simulink model "voltage_measure"  (R2025b)
settings: Solver=ode1be  StartTime=0.0  StopTime=simlength  FixedStep=ts  RelTol=1e-3
undefined symbols (not defined in the file): ts
libraries: fl_lib x36, nesl_utility x11, ee_lib x2, simulink x1
settings Model: Creator=ltnbda  LastModifiedBy=dbagn
settings DataIOCC: SaveOutput=off  SignalLogging=off  DSMLogging=off  SaveTime=off  ReturnWorkspaceOutputs=off
settings RTWCC: GPUComputeCapability=3.5

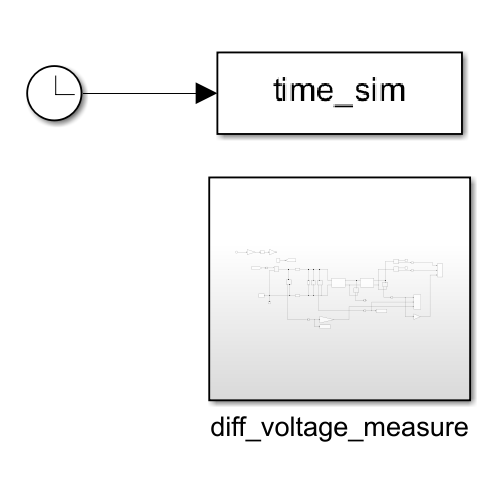
[thumbnail: Simulink's stored preview of the top-level diagram]
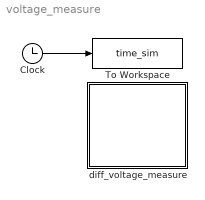
== system voltage_measure ==
  Clock : Clock
  To Workspace : ToWorkspace  VariableName=time_sim  SampleTime=ts
      settings: MaxDataPoints=N  Save2DSignal=2-D array (concatenate along first dimension)
  diff_voltage_measure : Subsystem
  wires:
  Clock/1 -> To Workspace/1

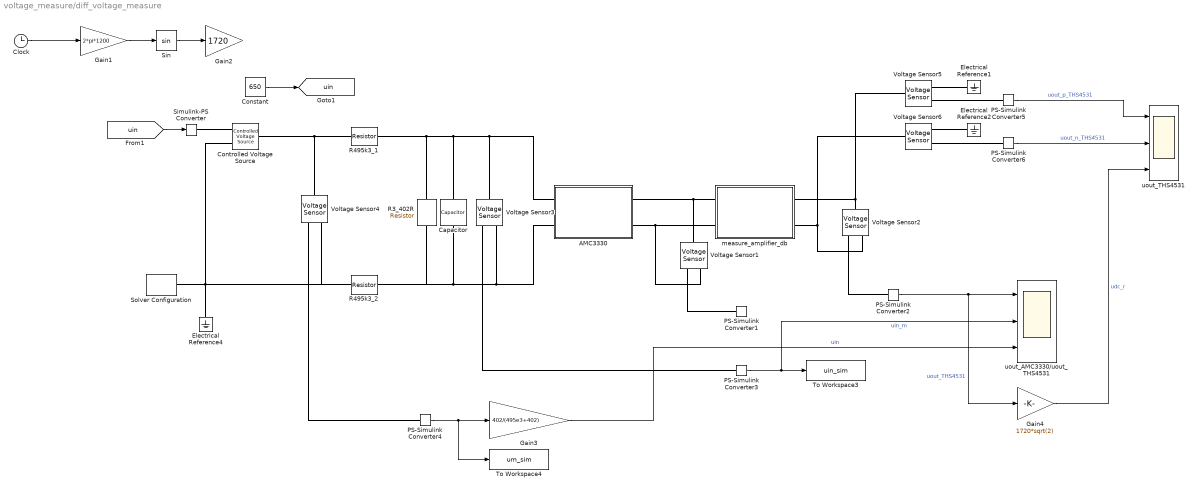
== system voltage_measure/diff_voltage_measure ==
  AMC3330 : Subsystem
  Capacitor : fl_lib/Electrical/Electrical Elements/Capacitor  c=0.1e-6 F  r=1e-6 Ohm  g=0 1/Ohm  i_specify=off  i_priority=None  i=0 A  i_nominal_specify=off  i_nominal_value=1  i_nominal_unit=A  v_specify=off  v_priority=None  v=0 V  v_nominal_specify=off  v_nominal_value=1  v_nominal_unit=V  vc_specify=off  vc_priority=High  vc=0 V  vc_nominal_specify=off  vc_nominal_value=1  vc_nominal_unit=V
  Clock : Clock
  Constant : Constant  Value=650
  Controlled Voltage Source : fl_lib/Electrical/Electrical Sources/Controlled Voltage Source
  Electrical Reference1 : fl_lib/Electrical/Electrical Elements/Electrical Reference
  Electrical Reference2 : fl_lib/Electrical/Electrical Elements/Electrical Reference
  Electrical Reference4 : fl_lib/Electrical/Electrical Elements/Electrical Reference
  Gain1 : Gain  Gain=2*pi*1200
  Gain2 : Gain  Gain=1720
  Gain3 : Gain  Gain=402/(495e3+402)
  Gain4 : Gain  Gain=1720*sqrt(2)
  PS-Simulink Converter{1..6} (6 alike) : nesl_utility/PS-Simulink Converter  PhysicalDomain=network_engine_domain  SubClassName=ps_output  LeftPortType=input  RightPortType=output  PseudoPeriodic=off  Frequencies=[]  VectorFormat=1-D array  Unit=V  AffineConversion=off
  R3_402R : fl_lib/Electrical/Electrical Elements/Resistor  R=402 Ohm  i_specify=off  i_priority=None  i=0 A  i_nominal_specify=off  i_nominal_value=1  i_nominal_unit=A  v_specify=off  v_priority=None  v=0 V  v_nominal_specify=off  v_nominal_value=1  v_nominal_unit=V
  R495k3_1 : fl_lib/Electrical/Electrical Elements/Resistor  R=400e3+95.3e3 Ohm  i_specify=off  i_priority=None  i=0 A  i_nominal_specify=off  i_nominal_value=1  i_nominal_unit=A  v_specify=off  v_priority=None  v=0 V  v_nominal_specify=off  v_nominal_value=1  v_nominal_unit=V
  R495k3_2 : fl_lib/Electrical/Electrical Elements/Resistor  R=400e3+95.3e3 Ohm  i_specify=off  i_priority=None  i=0 A  i_nominal_specify=off  i_nominal_value=1  i_nominal_unit=A  v_specify=off  v_priority=None  v=0 V  v_nominal_specify=off  v_nominal_value=1  v_nominal_unit=V
  Simulink-PS Converter : nesl_utility/Simulink-PS Converter  PhysicalDomain=network_engine_domain  SubClassName=ps_input  LeftPortType=input  RightPortType=output  PseudoPeriodic=off  Frequencies=[]  NoiseDistribution=none  NoiseParameters=[]  Unit=V  AffineConversion=off  FilteringAndDerivatives=provide  SimscapeFilterOrder=1  InputFilterTimeConstant=0.001  UdotUserProvided=0
  Sin : Trigonometry
  Solver Configuration : nesl_utility/Solver Configuration  PhysicalDomain=network_engine_domain  SubClassName=solver  LeftPortType=input  RightPortType=generic  Tones=[]  Harmonics=[]  SimulateNoise=off  Profile=off  UseLocalSampling=off  EnableSwitchedLinearOptims=on  FrequencyDomain=off  UseCCode=off  RelTol=0.001  AbsTol=0.001  MinStep=1e-09  ToWorkspace=off  RevertToSquareIcSolve=off  NumHomotopyIterations=100  PhasorMode=off  PhasorModeNumHarmonics=1  ConsistencySolver=NEWTON_XTOL_AFTER_FTOL  IndexReductionMethod=DerivativeReplacement  DoDC=on  ResidualTolerance=1e-09  ConsistencyTolSource=GLOBAL  ConsistencyAbsTol=0.001  ConsistencyRelTol=0.001  ConsistencyTolFactor=0.001  UseLocalSolver=on  LocalSolverChoice=NE_BACKWARD_EULER_ADVANCER  ResolveIndetEquations=on  FunctionEvalNumThread=1  LocalSolverSampleTime=ts  DoFixedCost=on  MaxNonlinIter=3  MaxModeIter=2  ComputeImpulses=off  ImpulseIterations=2  LinearAlgebra=auto  LinearAlgebraNumThread=0  EquationFormulation=NE_TIME_EF  DelaysMemoryBudget=1024  AutomaticFiltering=on  FilteringTimeConstant=0.001  PartitionStorageMethod=AS_NEEDED  PartitionMemoryBudget=1024  PartitionMethod=ROBUST  MultibodyUseLocalSolver=off  MultibodyLocalSolverChoice=ODE1  MultibodyLocalSolverSampleTime=0.001
  To Workspace3 : ToWorkspace  VariableName=uin_sim  SampleTime=ts
      settings: MaxDataPoints=N  Save2DSignal=2-D array (concatenate along first dimension)
  To Workspace4 : ToWorkspace  VariableName=um_sim  SampleTime=ts
      settings: MaxDataPoints=N  Save2DSignal=2-D array (concatenate along first dimension)
  Voltage Sensor{1..6} (6 alike) : fl_lib/Electrical/Electrical Sensors/Voltage Sensor
  measure_amplifier_db : Subsystem
  uout_AMC3330/uout_THS4531 : Scope  NumInputPorts=3
      settings: SampleTime=ts  ActiveDisplayYMinimum=0.26272599465267665  ActiveDisplayYMaximum=0.26382578383618316  DataLoggingVariableName=ScopeData2
  uout_THS4531 : Scope  NumInputPorts=3
      settings: ActiveDisplayString=3  ActiveDisplayYMinimum=582.121734260681  ActiveDisplayYMaximum=701.68902969605745  DataLoggingVariableName=ScopeData4
  tag scope: uin=global
  wires:
  PS-Simulink Converter2/1 -> uout_AMC3330/uout_THS4531/1, Gain4/1  "uout_THS4531"
  PS-Simulink Converter3/1 -> uout_AMC3330/uout_THS4531/2, To Workspace3/1  "uin_m"
  PS-Simulink Converter4/1 -> Gain3/1, To Workspace4/1
  [uin] -> Simulink-PS Converter/1
  Sin/1 -> Gain2/1
  Clock/1 -> Gain1/1
  Gain1/1 -> Sin/1
  Constant/1 -> [uin]
  PS-Simulink Converter5/1 -> uout_THS4531/1  "uout_p_THS4531"
  PS-Simulink Converter6/1 -> uout_THS4531/2  "uout_n_THS4531"
  Gain3/1 -> uout_AMC3330/uout_THS4531/3  "uin"
  Gain4/1 -> uout_THS4531/3  "udc_r"
  connections:
  R495k3_2/LConn1 -- Voltage Sensor4/RConn2 -- Controlled Voltage Source/RConn2 -- Solver Configuration/RConn1 -- Electrical Reference4/LConn1
  Controlled Voltage Source/LConn1 -- Voltage Sensor4/LConn1 -- R495k3_1/LConn1
  Simulink-PS Converter/RConn1 -- Controlled Voltage Source/RConn1
  R3_402R/LConn1 -- R495k3_1/RConn1 -- Capacitor/LConn1 -- Voltage Sensor3/LConn1 -- AMC3330/LConn1
  R495k3_2/RConn1 -- R3_402R/RConn1 -- Capacitor/RConn1 -- Voltage Sensor3/RConn2 -- AMC3330/LConn2
  AMC3330/RConn1 -- measure_amplifier_db/LConn1 -- Voltage Sensor1/LConn1
  Voltage Sensor2/LConn1 -- Voltage Sensor5/LConn1 -- measure_amplifier_db/RConn1
  Voltage Sensor2/RConn1 -- PS-Simulink Converter2/LConn1
  AMC3330/RConn2 -- Voltage Sensor1/RConn2 -- measure_amplifier_db/LConn2
  Voltage Sensor2/RConn2 -- Voltage Sensor6/LConn1 -- measure_amplifier_db/RConn2
  PS-Simulink Converter4/LConn1 -- Voltage Sensor4/RConn1
  Voltage Sensor3/RConn1 -- PS-Simulink Converter3/LConn1
  Voltage Sensor1/RConn1 -- PS-Simulink Converter1/LConn1
  Electrical Reference1/LConn1 -- Voltage Sensor5/RConn2
  Electrical Reference2/LConn1 -- Voltage Sensor6/RConn2
  PS-Simulink Converter5/LConn1 -- Voltage Sensor5/RConn1
  Voltage Sensor6/RConn1 -- PS-Simulink Converter6/LConn1

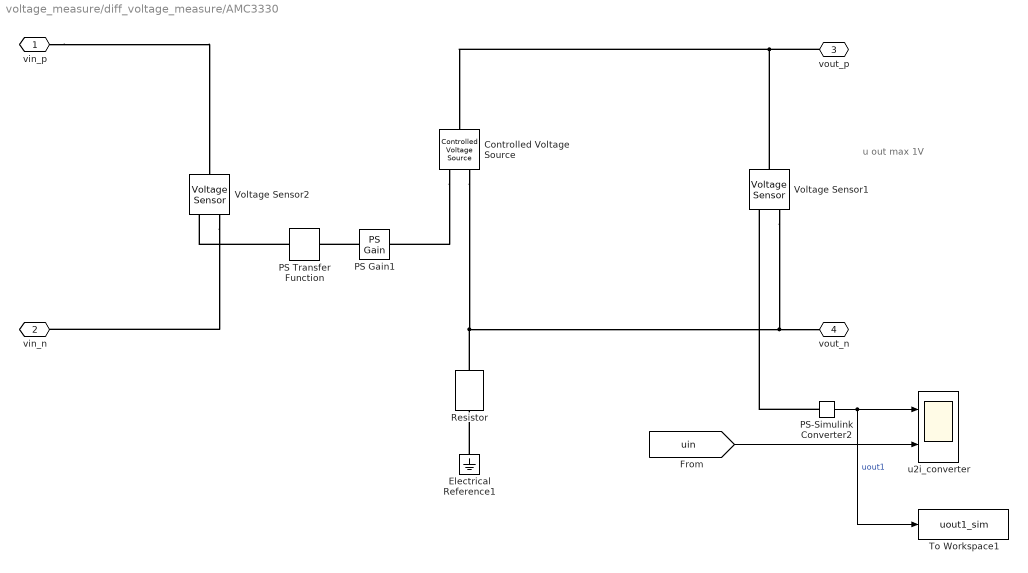
== system voltage_measure/diff_voltage_measure/AMC3330 ==
  note: u out max 1V
  Controlled Voltage Source : fl_lib/Electrical/Electrical Sources/Controlled Voltage Source
  Electrical Reference1 : fl_lib/Electrical/Electrical Elements/Electrical Reference
  PS Gain1 : fl_lib/Physical Signals/Functions/PS Gain  gain=2
  PS Transfer Function : fl_lib/Physical Signals/Linear Operators/PS Transfer Function  transfer_function_type=foundation.enum.transfer_function_type.lag  T=ts s  T1=2 s  T2=1 s  reset_method=foundation.enum.IntegratorResetSpec.None  initial_condition_spec=foundation.enum.IntegratorICSpec.Internal  y0=0 V
      settings: InternalSimscapePortConfiguration="{\"Bottom\":[],\"Left\":[{\"id\":\"U\",\"label\":\"\",\"type\":\"input\"}],\"Right\":[{\"id\":\"Y\",\"label\":\"\",\"type\":\"output\"}],\"Top\":[]}"
  PS-Simulink Converter2 : nesl_utility/PS-Simulink Converter  PhysicalDomain=network_engine_domain  SubClassName=ps_output  LeftPortType=input  RightPortType=output  PseudoPeriodic=off  Frequencies=[]  VectorFormat=1-D array  Unit=V  AffineConversion=off
  Resistor : fl_lib/Electrical/Electrical Elements/Resistor  R=1e6 Ohm  i_specify=off  i_priority=None  i=0 A  i_nominal_specify=off  i_nominal_value=1  i_nominal_unit=A  v_specify=off  v_priority=None  v=0 V  v_nominal_specify=off  v_nominal_value=1  v_nominal_unit=V
  To Workspace1 : ToWorkspace  VariableName=uout1_sim  SampleTime=ts
      settings: MaxDataPoints=N  Save2DSignal=2-D array (concatenate along first dimension)
  Voltage Sensor1 : fl_lib/Electrical/Electrical Sensors/Voltage Sensor
  Voltage Sensor2 : fl_lib/Electrical/Electrical Sensors/Voltage Sensor
  u2i_converter : Scope  NumInputPorts=2
      settings: SampleTime=ts  ActiveDisplayYMinimum=0.52734505076655569  ActiveDisplayYMaximum=0.52734505076682436
  vin_p : PMIOPort  Side=Left
  vin_n : PMIOPort  Port=2  Side=Left
  vout_p : PMIOPort  Port=3  Side=Right
  vout_n : PMIOPort  Port=4  Side=Right
  wires:
  [uin] -> u2i_converter/2
  PS-Simulink Converter2/1 -> To Workspace1/1, u2i_converter/1  "uout1"
  connections:
  vin_p/RConn1 -- Voltage Sensor2/LConn1
  Voltage Sensor2/RConn2 -- vin_n/RConn1
  PS Transfer Function/LConn1 -- Voltage Sensor2/RConn1
  Controlled Voltage Source/RConn1 -- PS Gain1/RConn1
  vout_p/RConn1 -- Controlled Voltage Source/LConn1 -- Voltage Sensor1/LConn1
  Controlled Voltage Source/RConn2 -- Resistor/LConn1 -- Voltage Sensor1/RConn2 -- vout_n/RConn1
  PS Gain1/LConn1 -- PS Transfer Function/RConn1
  PS-Simulink Converter2/LConn1 -- Voltage Sensor1/RConn1
  Electrical Reference1/LConn1 -- Resistor/RConn1

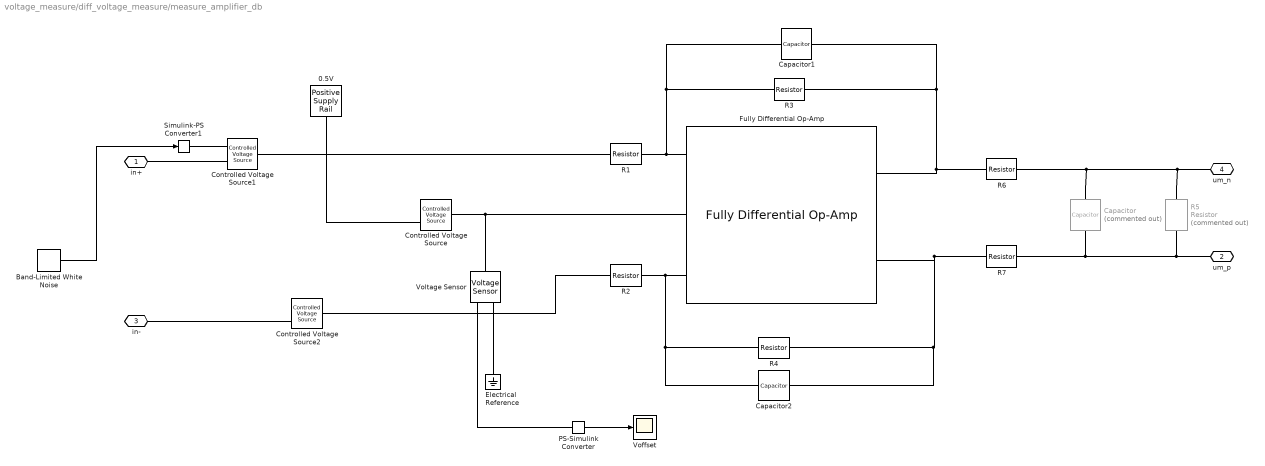
== system voltage_measure/diff_voltage_measure/measure_amplifier_db ==
  0.5V : ee_lib/Sources/Positive Supply Rail  v0=0.5 V
      settings: InternalSimscapePortConfiguration="{\"Bottom\":[],\"Left\":[],\"Right\":[{\"id\":\"p\",\"label\":\"\",\"type\":\"foundation.electrical.electrical\"}],\"Top\":[]}"
  Band-Limited White Noise : simulink/Sources/Band-Limited White Noise  Cov=1e-9  Ts=ts  seed=[23341]
  Capacitor : fl_lib/Electrical/Electrical Elements/Capacitor  Commented=on  c=22e-9 F  r=1e-6 Ohm  g=0 1/Ohm  i_specify=off  i_priority=None  i=0 A  i_nominal_specify=off  i_nominal_value=1  i_nominal_unit=A  v_specify=off  v_priority=None  v=0 V  v_nominal_specify=off  v_nominal_value=1  v_nominal_unit=V  vc_specify=off  vc_priority=High  vc=0 V  vc_nominal_specify=off  vc_nominal_value=1  vc_nominal_unit=V
  Capacitor1 : fl_lib/Electrical/Electrical Elements/Capacitor  c=5e-9 F  r=1e-6 Ohm  g=0 1/Ohm  i_specify=off  i_priority=None  i=0 A  i_nominal_specify=off  i_nominal_value=1  i_nominal_unit=A  v_specify=off  v_priority=None  v=0 V  v_nominal_specify=off  v_nominal_value=1  v_nominal_unit=V  vc_specify=off  vc_priority=High  vc=0 V  vc_nominal_specify=off  vc_nominal_value=1  vc_nominal_unit=V
  Capacitor2 : fl_lib/Electrical/Electrical Elements/Capacitor  c=5e-9 F  r=1e-6 Ohm  g=0 1/Ohm  i_specify=off  i_priority=None  i=0 A  i_nominal_specify=off  i_nominal_value=1  i_nominal_unit=A  v_specify=off  v_priority=None  v=0 V  v_nominal_specify=off  v_nominal_value=1  v_nominal_unit=V  vc_specify=off  vc_priority=High  vc=0 V  vc_nominal_specify=off  vc_nominal_value=1  vc_nominal_unit=V
  Controlled Voltage Source : fl_lib/Electrical/Electrical Sources/Controlled Voltage Source
  Controlled Voltage Source1 : fl_lib/Electrical/Electrical Sources/Controlled Voltage Source
  Controlled Voltage Source2 : fl_lib/Electrical/Electrical Sources/Controlled Voltage Source
  Electrical Reference : fl_lib/Electrical/Electrical Elements/Electrical Reference
  Fully Differential Op-Amp : ee_lib/Integrated Circuits/Fully Differential Op-Amp  A=1e3  f=1.5 GHz  Rdiff=1.3 MOhm  Cdiff=1.8 pF  Rcom=1.0 MOhm  Ccom=2.3 pF  Rout=1 Ohm  Vmin=-1.4 V  Vmax=1.4 V  Vdotdiff=5000 V/us  Rocm=23.0 kOhm  Vs_neg=-5 V  Vs_pos=5 V  V0=0 V
      settings: InternalSimscapePortConfiguration="{\"Bottom\":[],\"Left\":[{\"id\":\"n\",\"label\":\"-\",\"type\":\"foundation.electrical.electrical\"},{\"id\":\"cm\",\"label\":\"cm\",\"type\":\"foundation.electrical.electrical\"},{\"id\":\"p\",\"label\":\"+\",\"type\":\"foundation.electrical.electrical\"}],\"Right\":[{\"id\":\"out_p\",\"label\":\"+\",\"type\":\"foundation.electrical.electrical\"},{\"id\":\"out_n\",\"label\":\"-\",\"type\":\"foundation.electrical.electrical\"}],\"Top\":[]}"
  PS-Simulink Converter : nesl_utility/PS-Simulink Converter  PhysicalDomain=network_engine_domain  SubClassName=ps_output  LeftPortType=input  RightPortType=output  PseudoPeriodic=off  Frequencies=[]  VectorFormat=1-D array  Unit=V  AffineConversion=off
  R1 : fl_lib/Electrical/Electrical Elements/Resistor  R=2e3 Ohm  i_specify=off  i_priority=None  i=0 A  i_nominal_specify=off  i_nominal_value=1  i_nominal_unit=A  v_specify=off  v_priority=None  v=0 V  v_nominal_specify=off  v_nominal_value=1  v_nominal_unit=V
  R2 : fl_lib/Electrical/Electrical Elements/Resistor  R=2e3 Ohm  i_specify=off  i_priority=None  i=0 A  i_nominal_specify=off  i_nominal_value=1  i_nominal_unit=A  v_specify=off  v_priority=None  v=0 V  v_nominal_specify=off  v_nominal_value=1  v_nominal_unit=V
  R3 : fl_lib/Electrical/Electrical Elements/Resistor  R=1e3 Ohm  i_specify=off  i_priority=None  i=0 A  i_nominal_specify=off  i_nominal_value=1  i_nominal_unit=A  v_specify=off  v_priority=None  v=0 V  v_nominal_specify=off  v_nominal_value=1  v_nominal_unit=V
  R4 : fl_lib/Electrical/Electrical Elements/Resistor  R=1e3 Ohm  i_specify=off  i_priority=None  i=0 A  i_nominal_specify=off  i_nominal_value=1  i_nominal_unit=A  v_specify=off  v_priority=None  v=0 V  v_nominal_specify=off  v_nominal_value=1  v_nominal_unit=V
  R5 : fl_lib/Electrical/Electrical Elements/Resistor  Commented=on  R=2e3 Ohm  i_specify=off  i_priority=None  i=0 A  i_nominal_specify=off  i_nominal_value=1  i_nominal_unit=A  v_specify=off  v_priority=None  v=0 V  v_nominal_specify=off  v_nominal_value=1  v_nominal_unit=V
  R6 : fl_lib/Electrical/Electrical Elements/Resistor  R=150 Ohm  i_specify=off  i_priority=None  i=0 A  i_nominal_specify=off  i_nominal_value=1  i_nominal_unit=A  v_specify=off  v_priority=None  v=0 V  v_nominal_specify=off  v_nominal_value=1  v_nominal_unit=V
  R7 : fl_lib/Electrical/Electrical Elements/Resistor  R=150 Ohm  i_specify=off  i_priority=None  i=0 A  i_nominal_specify=off  i_nominal_value=1  i_nominal_unit=A  v_specify=off  v_priority=None  v=0 V  v_nominal_specify=off  v_nominal_value=1  v_nominal_unit=V
  Simulink-PS Converter1 : nesl_utility/Simulink-PS Converter  PhysicalDomain=network_engine_domain  SubClassName=ps_input  LeftPortType=input  RightPortType=output  PseudoPeriodic=off  Frequencies=[]  NoiseDistribution=none  NoiseParameters=[]  Unit=V  AffineConversion=off  FilteringAndDerivatives=provide  SimscapeFilterOrder=1  InputFilterTimeConstant=0.001  UdotUserProvided=0
  Voffset : Scope
      settings: SampleTime=ts  ActiveDisplayYMinimum=-0.059473389598419614  ActiveDisplayYMaximum=1.0507912739067826
  Voltage Sensor : fl_lib/Electrical/Electrical Sensors/Voltage Sensor
  in+ : PMIOPort  Side=Left
  um_p : PMIOPort  Port=2  Side=Right
  in- : PMIOPort  Port=3  Side=Left
  um_n : PMIOPort  Port=4  Side=Right
  wires:
  Band-Limited White Noise/1 -> Simulink-PS Converter1/1
  PS-Simulink Converter/1 -> Voffset/1
  connections:
  R3/RConn1 -- Capacitor1/RConn1 -- R6/LConn1 -- Fully Differential Op-Amp/RConn2
  R4/RConn1 -- Capacitor2/RConn1 -- Fully Differential Op-Amp/RConn1 -- R7/LConn1
  R6/RConn1 -- Capacitor/LConn1 -- R5/LConn1 -- um_n/RConn1
  R7/RConn1 -- Capacitor/RConn1 -- R5/RConn1 -- um_p/RConn1
  Controlled Voltage Source/LConn1 -- Voltage Sensor/LConn1 -- Fully Differential Op-Amp/LConn2
  0.5V/RConn1 -- Controlled Voltage Source/RConn2
  Fully Differential Op-Amp/LConn1 -- R2/RConn1 -- Capacitor2/LConn1 -- R4/LConn1
  PS-Simulink Converter/LConn1 -- Voltage Sensor/RConn1
  Electrical Reference/LConn1 -- Voltage Sensor/RConn2
  R1/RConn1 -- R3/LConn1 -- Capacitor1/LConn1 -- Fully Differential Op-Amp/LConn3
  in+/RConn1 -- Controlled Voltage Source1/RConn2
  Controlled Voltage Source1/LConn1 -- R1/LConn1
  Simulink-PS Converter1/RConn1 -- Controlled Voltage Source1/RConn1
  in-/RConn1 -- Controlled Voltage Source2/RConn2
  Controlled Voltage Source2/LConn1 -- R2/LConn1
